simulink model "tuning_artigo"  (R2017a)
settings: Solver=VariableStepAuto  StartTime=0.0  StopTime=1000  RelTol=1e-3
undefined symbols (not defined in the file or in its folder): magnitude
libraries: simulink x1
settings Model: Creator=filip  LastModifiedBy=filip

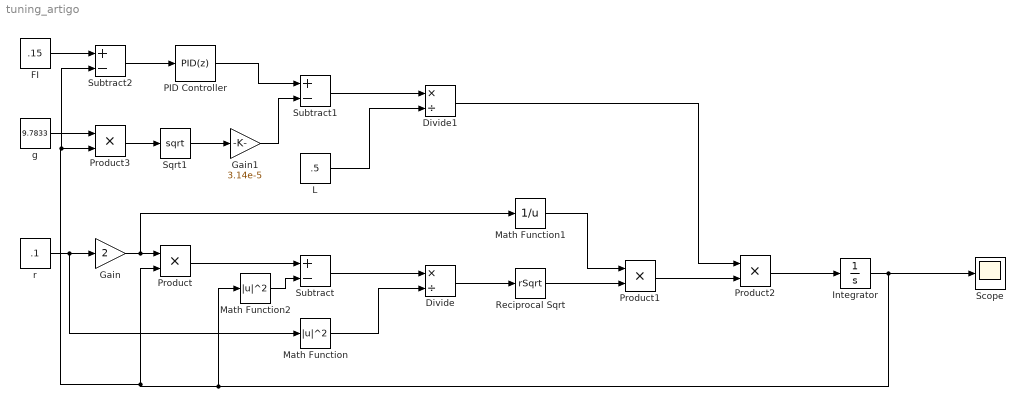
== system tuning_artigo ==
  Divide : Product  Inputs=*/
  Divide1 : Product  Inputs=*/
  FI : Constant  Value=.15
  Gain : Gain  Gain=2
  Gain1 : Gain  Gain=3.14e-5
  Integrator : Integrator  InitialCondition=.1
  L : Constant  Value=.5
  Math Function : Math  Operator=magnitude^2  SaturateOnIntegerOverflow=on
  Math Function1 : Math  Operator=reciprocal  SaturateOnIntegerOverflow=on
  Math Function2 : Math  Operator=magnitude^2  SaturateOnIntegerOverflow=on
  PID Controller : simulink/Continuous/PID Controller  Controller=PID  TimeDomain=Discrete-time  SampleTime=1  IntegratorMethod=Forward Euler  FilterMethod=Forward Euler  Form=Parallel  UseFilter=off  ControllerParametersSource=internal  P=0.00276655231239209  I=2.01221674060025e-05  D=0.00137824561434454  N=0.182730079681475  InitialConditionSource=internal  InitialConditionForIntegrator=0  InitialConditionForFilter=0  ExternalReset=none  LimitOutput=off  UpperSaturationLimit=inf  LowerSaturationLimit=-inf  LinearizeAsGain=on  AntiWindupMode=none  Kb=1  TrackingMode=off  Kt=1  PParamMin=[]  PParamMax=[]  IParamMin=[]  IParamMax=[]  DParamMin=[]  DParamMax=[]  NParamMin=[]  NParamMax=[]  KbParamMin=[]  KbParamMax=[]  KtParamMin=[]  KtParamMax=[]  POutMin=[]  POutMax=[]  IOutMin=[]  IOutMax=[]  DOutMin=[]  DOutMax=[]  NOutMin=[]  NOutMax=[]  KbOutMin=[]  KbOutMax=[]  KtOutMin=[]  KtOutMax=[]  IntegratorOutMin=[]  IntegratorOutMax=[]  FilterOutMin=[]  FilterOutMax=[]  SumOutMin=[]  SumOutMax=[]  SumI1OutMin=[]  SumI1OutMax=[]  SumI2OutMin=[]  SumI2OutMax=[]  SumI3OutMin=[]  SumI3OutMax=[]  SumDOutMin=[]  SumDOutMax=[]  SaturationOutMin=[]  SaturationOutMax=[]  IntegratorContinuousStateAttributes=''  IntegratorStateMustResolveToSignalObject=off  IntegratorRTWStateStorageClass=Auto  FilterContinuousStateAttributes=''  FilterStateMustResolveToSignalObject=off  FilterRTWStateStorageClass=Auto  DifferentiatorICPrevScaledInput=0  DifferentiatorOutMin=[]  DifferentiatorOutMax=[]  InitialConditionSetting=State (most efficient)
  Product{,1..3} (4 alike) : Product
  Reciprocal Sqrt : Sqrt  Operator=rSqrt  SaturateOnIntegerOverflow=on
  Scope : Scope
  Sqrt1 : Sqrt  SaturateOnIntegerOverflow=on
  Subtract : Sum  Inputs=+-
  Subtract1 : Sum  Inputs=+-
  Subtract2 : Sum  Inputs=+-
  g : Constant  Value=9.7833
  r : Constant  Value=.1
  wires:
  r/1 -> Math Function/1, Gain/1
  Product/1 -> Subtract/1
  Gain/1 -> Math Function1/1, Product/1
  Subtract/1 -> Divide/1
  Math Function/1 -> Divide/2
  Divide/1 -> Reciprocal Sqrt/1
  Reciprocal Sqrt/1 -> Product1/2
  Math Function1/1 -> Product1/1
  Product1/1 -> Product2/2
  Sqrt1/1 -> Gain1/1
  g/1 -> Product3/1
  Product3/1 -> Sqrt1/1
  Gain1/1 -> Subtract1/2
  Subtract1/1 -> Divide1/1
  L/1 -> Divide1/2
  Divide1/1 -> Product2/1
  Product2/1 -> Integrator/1
  Integrator/1 -> Scope/1, Math Function2/1, Subtract2/2, Product3/2, Product/2
  Math Function2/1 -> Subtract/2
  FI/1 -> Subtract2/1
  Subtract2/1 -> PID Controller/1
  PID Controller/1 -> Subtract1/1
